simulink library "tqen"  (Simulink 8.2)
settings: Solver=ode45  SolverMode=SingleTasking  StartTime=0.0  StopTime=10.0  RelTol=1e-3
undefined symbols (not defined in the file or in its folder): ATQEN_BaseBrkDerateRatD_X_pct, ATQEN_BaseVehSpdRatD_X_kph, ATQEN_CruzAccLimIMult_X_mps2, ATQEN_CruzAccLimPMult_X_mps2, ATQEN_CruzContIMult_X_kph, ATQEN_CruzContPMult_X_kph, ATQEN_EngTqBrkMap_X_erpm, C_TASK_5MS_S, C_TICK_TIME_S, ENUM_ECMTQSOURCE_EXTERNAL, ENUM_ECMTQSOURCE_INTERNAL, ENUM_ECMTQSOURCE_TORQUELIM, ENUM_EMSHYBRIDOPSTATE_HYBRIDENABLE, ENUM_EMSOPSTATE_NORMAL, ENUM_GEARPOSN_PN, FALSE, KTQEN_AccelPedalFiltTm_s, KTQEN_BrakeSWTqDsblTimeThres_s, KTQEN_CruzAccLimErrGain_rat, KTQEN_CruzAccLimIGain_rat, KTQEN_CruzAccLimIMax_Nm, KTQEN_CruzAccLimIMin_Nm, KTQEN_CruzAccLimIRest_flg, KTQEN_CruzAccLimPGain_rat, KTQEN_CruzContAccLim_G, KTQEN_CruzContAccLimTqMax_Nm, KTQEN_CruzContAccLimTqMin_Nm, KTQEN_CruzContEnblSW_flg, KTQEN_CruzContErrGain_rat, KTQEN_CruzContIGain_rat, KTQEN_CruzContIMax_Nm, KTQEN_CruzContIMin_Nm, KTQEN_CruzContIRest_flg, KTQEN_CruzContPGain_rat, KTQEN_CruzContResumeSW_flg, KTQEN_CruzContSetSW_flg, KTQEN_CruzDsblDefaultTq_Nm, KTQEN_CruzSpdChgTimeThres_s, KTQEN_CruzTgSpdSetFalRate_kphps, KTQEN_CruzTgSpdSetRisRate_kphps, KTQEN_EngBrkTqMaxOvrd_Nm, KTQEN_EngBrkTqMinOvrd_Nm, KTQEN_VehAccCalRate_s, KTQEN_VehAccFltConst_s, KTQEN_VehSpdMaxVal_kph, KTQEN_VSGOVErrGain_rat, KTQEN_VSGOVIGain_rat, KTQEN_VSGOVIMax_Nm, KTQEN_VSGOVIMin_Nm, KTQEN_VSGOVIRest_flg, KTQEN_VSGOVMinVehSpd_kph, KTQEN_VSGOVPGain_rat, KTQEN_VSGOVTqDefault_Nm, KTQEN_VSGOVTqMax_Nm, KTQEN_VSGOVTqMin_Nm, MTQEN_BaseBrkDerateRatD_Y_pct, MTQEN_BasePedalSportMapHiSpdD_Z_pct, MTQEN_BasePedalSportMapLoSpdD_Z_pct, MTQEN_BaseTqSupptDeltPdlD_X_pctps, MTQEN_BaseTqSupptDeltPdlD_Y_pct ... (+9)
libraries: hcu_lib x6, tqen x3, simulink x1
(part 2 of 2)

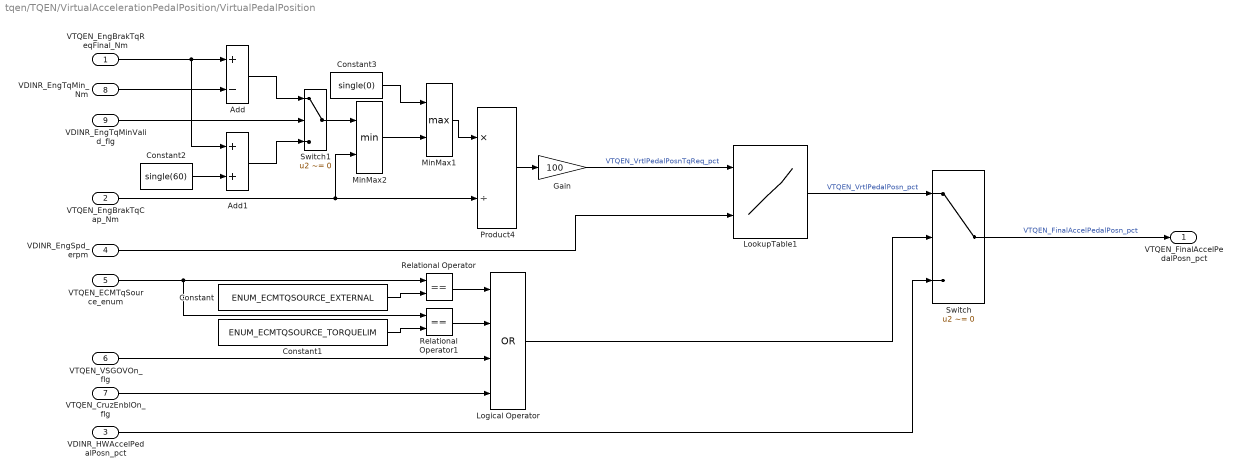
== system tqen/TQEN/VirtualAccelerationPedalPosition/VirtualPedalPosition ==
  VTQEN_EngBrakTqReqFinal_Nm : Inport
  VTQEN_EngBrakTqCap_Nm : Inport  Port=2
  VDINR_HWAccelPedalPosn_pct : Inport  Port=3
  VDINR_EngSpd_erpm : Inport  Port=4
  VTQEN_ECMTqSource_enum : Inport  Port=5
  VTQEN_VSGOVOn_flg : Inport  Port=6
  VTQEN_CruzEnblOn_flg : Inport  Port=7
  VDINR_EngTqMin_Nm : Inport  Port=8
  VDINR_EngTqMinValid_flg : Inport  Port=9
  Add : Sum  Inputs=+-
  Add1 : Sum
  Constant : Constant  Value=ENUM_ECMTQSOURCE_EXTERNAL
  Constant1 : Constant  Value=ENUM_ECMTQSOURCE_TORQUELIM
  Constant2 : Constant  Value=single(60)
  Constant3 : Constant  Value=single(0)
  Gain : Gain  Gain=100
  Logical Operator : Logic  Operator=OR  Inputs=4  AllPortsSameDT=off  OutDataTypeStr=boolean
  LookupTable1 : Lookup2D  RowIndex=ATQEN_VirtualPedalMap_X_pct  ColumnIndex=ATQEN_VirtualPedalMap_Y_erpm  Table=MTQEN_VirtualPedalMap_Z_pct  LookUpMeth=Interpolation-Use End Values
      settings: AttributesFormatString=<row =%<RowIndex>>\n<column = %<ColumnIndex>>\n<output = %<Table>>
  MinMax1 : MinMax  Function=max  Inputs=2
  MinMax2 : MinMax  Inputs=2
  Product4 : Product  Inputs=*/  RndMeth=Zero
  Relational Operator : RelationalOperator  Operator===  OutDataTypeStr=boolean
  Relational Operator1 : RelationalOperator  Operator===  OutDataTypeStr=boolean
  Switch : Switch  Criteria=u2 ~= 0
  Switch1 : Switch  Criteria=u2 ~= 0
  VTQEN_FinalAccelPedalPosn_pct : Outport
  wires:
  Constant3/1 -> MinMax1/1
  MinMax2/1 -> MinMax1/2
  Constant2/1 -> Add1/2
  VTQEN_EngBrakTqReqFinal_Nm/1 -> Add/1, Add1/1
  Add1/1 -> Switch1/3
  VDINR_EngTqMinValid_flg/1 -> Switch1/2
  Switch1/1 -> MinMax2/1
  VDINR_EngTqMin_Nm/1 -> Add/2
  Add/1 -> Switch1/1
  VTQEN_CruzEnblOn_flg/1 -> Logical Operator/4
  VTQEN_VSGOVOn_flg/1 -> Logical Operator/3
  Constant1/1 -> Relational Operator1/2
  Relational Operator1/1 -> Logical Operator/2
  Constant/1 -> Relational Operator/2
  Logical Operator/1 -> Switch/2
  LookupTable1/1 -> Switch/1  "VTQEN_VrtlPedalPosn_pct"
  VDINR_EngSpd_erpm/1 -> LookupTable1/2
  Relational Operator/1 -> Logical Operator/1
  Gain/1 -> LookupTable1/1  "VTQEN_VrtlPedalPosnTqReq_pct"
  Product4/1 -> Gain/1
  VTQEN_EngBrakTqCap_Nm/1 -> Product4/2, MinMax2/2
  MinMax1/1 -> Product4/1
  VDINR_HWAccelPedalPosn_pct/1 -> Switch/3
  VTQEN_ECMTqSource_enum/1 -> Relational Operator1/1, Relational Operator/1
  Switch/1 -> VTQEN_FinalAccelPedalPosn_pct/1  "VTQEN_FinalAccelPedalPosn_pct"

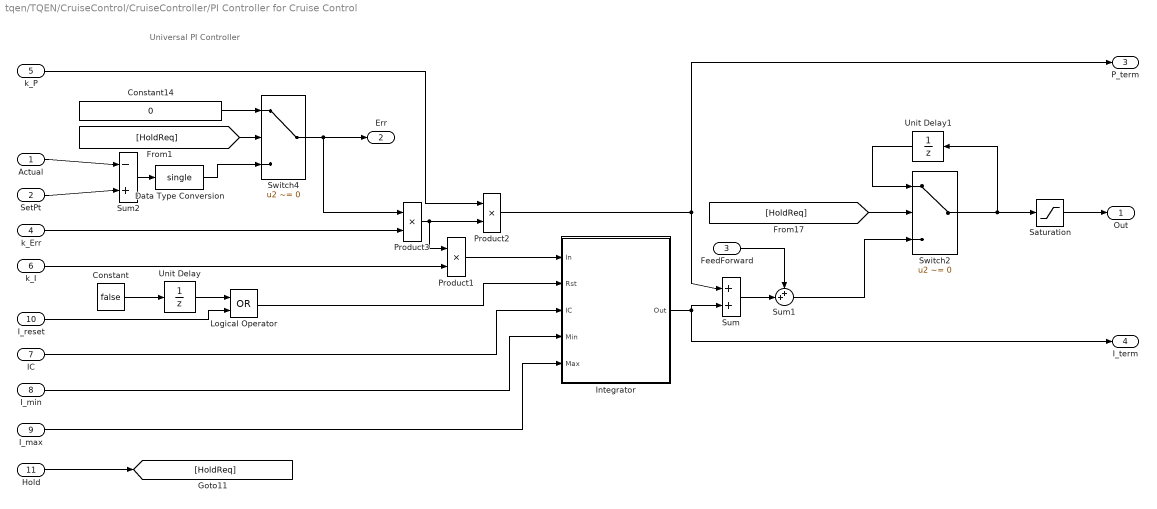
== system tqen/TQEN/CruiseControl/CruiseController/PI Controller for Cruise Control ==
  note: Universal PI Controller
  Actual : Inport
  SetPt : Inport  Port=2
  FeedForward : Inport  Port=3
  k_Err : Inport  Port=4
  k_P : Inport  Port=5
  k_I : Inport  Port=6
  IC : Inport  Port=7
  I_min : Inport  Port=8
  I_max : Inport  Port=9
  I_reset : Inport  Port=10
  Hold : Inport  Port=11
  Constant : Constant  Value=false  OutDataTypeStr=boolean
  Constant14 : Constant  Value=0  OutDataTypeStr=single
  Data Type Conversion : DataTypeConversion  OutDataTypeStr=single  SaturateOnIntegerOverflow=on  RndMeth=Zero
  Integrator : Subsystem  TreatAsAtomicUnit=on
  Logical Operator : Logic  Operator=OR  AllPortsSameDT=off  OutDataTypeStr=boolean
  Product1 : Product  InputSameDT=on  OutDataTypeStr=Inherit: Same as first input
  Product2 : Product  InputSameDT=on  OutDataTypeStr=Inherit: Same as first input
  Product3 : Product  InputSameDT=on  OutDataTypeStr=Inherit: Same as first input
  Saturation : Saturate  UpperLimit=inf  LowerLimit=0
  Sum : Sum  Inputs=+|+  SaturateOnIntegerOverflow=on  InputSameDT=on  OutDataTypeStr=Inherit: Same as first input
  Sum1 : Sum  Inputs=++|
  Sum2 : Sum  Inputs=-|+  SaturateOnIntegerOverflow=on  InputSameDT=on  OutDataTypeStr=Inherit: Same as first input
  Switch2 : Switch  Criteria=u2 ~= 0
  Switch4 : Switch  Criteria=u2 ~= 0
  Unit Delay : UnitDelay  InitialCondition=true  SampleTime=-1
  Unit Delay1 : UnitDelay  SampleTime=-1
  Out : Outport  OutputWhenDisabled=reset  InitialOutput=[0]
  Err : Outport  Port=2  OutputWhenDisabled=reset  InitialOutput=[0]
  P_term : Outport  Port=3  OutputWhenDisabled=reset  InitialOutput=[0]
  I_term : Outport  Port=4  OutputWhenDisabled=reset  InitialOutput=[0]
  wires:
  I_max/1 -> Integrator/5(Max)
  I_min/1 -> Integrator/4(Min)
  k_Err/1 -> Product3/2
  SetPt/1 -> Sum2/2
  Actual/1 -> Sum2/1
  k_P/1 -> Product2/1
  k_I/1 -> Product1/2
  Product1/1 -> Integrator/1(In)
  Product2/1 -> P_term/1, Sum/1
  Integrator/1(Out) -> I_term/1, Sum/2
  Sum/1 -> Sum1/2
  IC/1 -> Integrator/3(IC)
  Product3/1 -> Product2/2, Product1/1
  Sum2/1 -> Data Type Conversion/1
  Logical Operator/1 -> Integrator/2(Rst)
  I_reset/1 -> Logical Operator/2
  Unit Delay/1 -> Logical Operator/1
  Constant/1 -> Unit Delay/1
  Hold/1 -> [HoldReq]
  [HoldReq] -> Switch2/2
  Switch2/1 -> Unit Delay1/1, Saturation/1
  Unit Delay1/1 -> Switch2/1
  Switch4/1 -> Err/1, Product3/1
  Data Type Conversion/1 -> Switch4/3
  [HoldReq] -> Switch4/2
  Constant14/1 -> Switch4/1
  Sum1/1 -> Switch2/3
  FeedForward/1 -> Sum1/1
  Saturation/1 -> Out/1

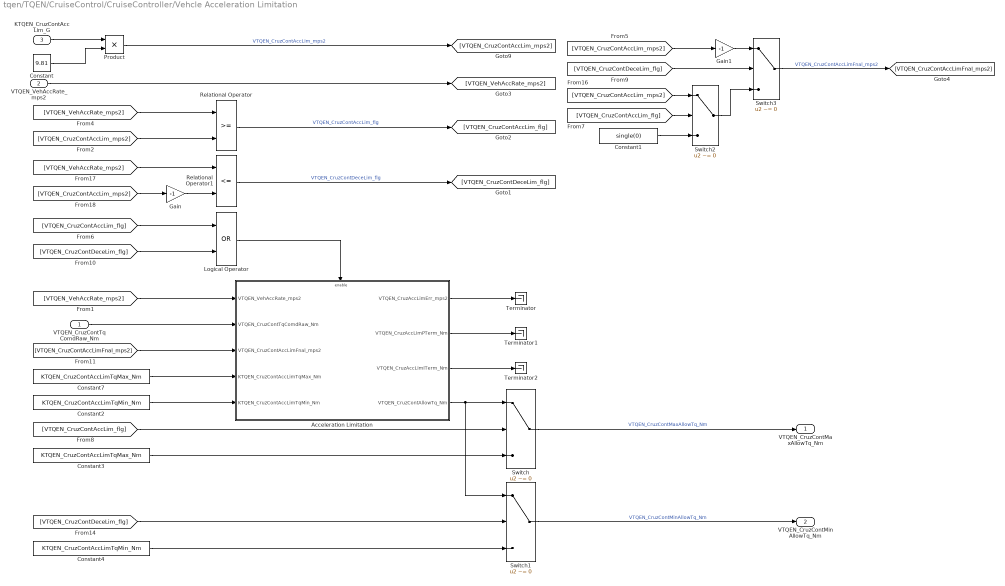
== system tqen/TQEN/CruiseControl/CruiseController/Vehcle Acceleration Limitation ==
  VTQEN_CruzContTqComdRaw_Nm : Inport
  VTQEN_VehAccRate_mps2 : Inport  Port=2
  KTQEN_CruzContAccLim_G : Inport  Port=3
  Acceleration Limitation : Subsystem  TreatAsAtomicUnit=on
  Constant : Constant  Value=9.81  OutDataTypeStr=single
  Constant1 : Constant  Value=single(0)
  Constant2 : Constant  Value=KTQEN_CruzContAccLimTqMin_Nm
  Constant3 : Constant  Value=KTQEN_CruzContAccLimTqMax_Nm
  Constant4 : Constant  Value=KTQEN_CruzContAccLimTqMin_Nm
  Constant7 : Constant  Value=KTQEN_CruzContAccLimTqMax_Nm
  Gain : Gain  Gain=-1
  Gain1 : Gain  Gain=-1
  Logical Operator : Logic  Operator=OR  AllPortsSameDT=off  OutDataTypeStr=boolean
  Product : Product  RndMeth=Zero
  Relational Operator : RelationalOperator  OutDataTypeStr=boolean
  Relational Operator1 : RelationalOperator  Operator=<=  OutDataTypeStr=boolean
  Switch{,1..3} (4 alike) : Switch  Criteria=u2 ~= 0
  Terminator : Terminator
  Terminator1 : Terminator
  Terminator2 : Terminator
  VTQEN_CruzContMaxAllowTq_Nm : Outport
  VTQEN_CruzContMinAllowTq_Nm : Outport  Port=2
  wires:
  Acceleration Limitation/3(VTQEN_CruzAccLimITerm_Nm) -> Terminator2/1
  Acceleration Limitation/2(VTQEN_CruzAccLimPTerm_Nm) -> Terminator1/1
  Constant2/1 -> Acceleration Limitation/5(KTQEN_CruzContAccLimTqMin_Nm)
  [VTQEN_CruzContDeceLim_flg] -> Logical Operator/2
  [VTQEN_CruzContAccLim_flg] -> Logical Operator/1
  Switch3/1 -> [VTQEN_CruzContAccLimFnal_mps2]  "VTQEN_CruzContAccLimFnal_mps2"
  Gain1/1 -> Switch3/1
  [VTQEN_CruzContAccLim_mps2] -> Gain1/1
  Switch2/1 -> Switch3/3
  [VTQEN_CruzContDeceLim_flg] -> Switch3/2
  Constant1/1 -> Switch2/3
  [VTQEN_CruzContAccLim_mps2] -> Switch2/1
  [VTQEN_CruzContAccLim_flg] -> Switch2/2
  Constant7/1 -> Acceleration Limitation/4(KTQEN_CruzContAccLimTqMax_Nm)
  [VTQEN_CruzContDeceLim_flg] -> Switch1/2
  [VTQEN_CruzContAccLim_flg] -> Switch/2
  Constant4/1 -> Switch1/3
  Switch1/1 -> VTQEN_CruzContMinAllowTq_Nm/1  "VTQEN_CruzContMinAllowTq_Nm"
  Gain/1 -> Relational Operator1/2
  Relational Operator1/1 -> [VTQEN_CruzContDeceLim_flg]  "VTQEN_CruzContDeceLim_flg"
  [VTQEN_CruzContAccLim_mps2] -> Gain/1
  [VTQEN_VehAccRate_mps2] -> Relational Operator1/1
  Relational Operator/1 -> [VTQEN_CruzContAccLim_flg]  "VTQEN_CruzContAccLim_flg"
  [VTQEN_CruzContAccLim_mps2] -> Relational Operator/2
  [VTQEN_VehAccRate_mps2] -> Relational Operator/1
  VTQEN_VehAccRate_mps2/1 -> [VTQEN_VehAccRate_mps2]
  Constant/1 -> Product/2
  KTQEN_CruzContAccLim_G/1 -> Product/1
  Product/1 -> [VTQEN_CruzContAccLim_mps2]  "VTQEN_CruzContAccLim_mps2"
  Logical Operator/1 -> Acceleration Limitation/Enable
  Constant3/1 -> Switch/3
  Acceleration Limitation/4(VTQEN_CruzContAllowTq_Nm) -> Switch1/1, Switch/1
  [VTQEN_VehAccRate_mps2] -> Acceleration Limitation/1(VTQEN_VehAccRate_mps2)
  VTQEN_CruzContTqComdRaw_Nm/1 -> Acceleration Limitation/2(VTQEN_CruzContTqComdRaw_Nm)
  [VTQEN_CruzContAccLimFnal_mps2] -> Acceleration Limitation/3(VTQEN_CruzContAccLimFnal_mps2)
  Switch/1 -> VTQEN_CruzContMaxAllowTq_Nm/1  "VTQEN_CruzContMaxAllowTq_Nm"
  Acceleration Limitation/1(VTQEN_CruzAccLimErr_mps2) -> Terminator/1

== system tqen/TQEN/CruiseControl/Rate_Limit/RateLimiter ==
  Data_Input : Inport
  Rising Rate : Inport  Port=2
  Falling Rate : Inport  Port=3
  Initial_Condition : Inport  Port=4
  Chart : Stateflow chart  TreatAsAtomicUnit=on
  Constant : Constant  Value=C_TICK_TIME_S
  Constant1 : Constant  Value=C_TICK_TIME_S
  Constant2 : Constant  Value=single(1)
  Constant4 : Constant  Value=single(1)
  Data Type Conversion : DataTypeConversion  OutDataTypeStr=boolean
  Data Type Conversion1 : DataTypeConversion  OutDataTypeStr=boolean
  Product{1..4} (4 alike) : Product  Inputs=*/  RndMeth=Zero
  Relational Operator : RelationalOperator  Operator=>  OutDataTypeStr=boolean
  Relational Operator1 : RelationalOperator  Operator=<  OutDataTypeStr=boolean
  Saturation : Subsystem
  Sum1 : Sum  Inputs=|++
  Switch1 : Switch  Threshold=0.5
  Unit Delay1 : UnitDelay  SampleTime=-1
  Data_Output : Outport
  wires:
  Constant2/1 -> Product4/1
  Unit Delay1/1 -> Relational Operator1/2, Relational Operator/2, Sum1/2
  Sum1/1 -> Saturation/1(in)
  Falling Rate/1 -> Product2/1
  Rising Rate/1 -> Product1/1
  Switch1/1 -> Unit Delay1/1, Data_Output/1
  Constant1/1 -> Product4/2
  Constant4/1 -> Product3/1
  Constant/1 -> Product3/2
  Initial_Condition/1 -> Switch1/1
  Chart/1(Initial) -> Switch1/2
  Chart/4(Max) -> Saturation/3(max)
  Chart/3(Min) -> Saturation/2(min)
  Saturation/1(out) -> Switch1/3
  Chart/2(tou) -> Sum1/1
  Data Type Conversion1/1 -> Chart/1(increase)
  Data Type Conversion/1 -> Chart/2(decrease)
  Product2/1 -> Chart/5(decrease_tou)
  Product1/1 -> Chart/4(increase_tou)
  Product4/1 -> Product2/2
  Product3/1 -> Product1/2
  Data_Input/1 -> Chart/3(Data_in), Relational Operator1/1, Relational Operator/1
  Relational Operator/1 -> Data Type Conversion1/1
  Relational Operator1/1 -> Data Type Conversion/1

== system tqen/TQEN/CruiseControl/Trigger signal generator/trigger signal generator ==
  Time_dur [s] : Inport
  Constant3 : Constant  Value=0  OutDataTypeStr=single
  Constant4 : Constant  Value=C_TICK_TIME_S
  Relational Operator1 : RelationalOperator  OutDataTypeStr=boolean
  Sum1 : Sum  Inputs=|++  SaturateOnIntegerOverflow=on  InputSameDT=on
  Sum2 : Sum  Inputs=+-
  Switch3 : Switch  Threshold=0.5
  Unit Delay2 : UnitDelay  SampleTime=-1
  Unit Delay3 : UnitDelay  SampleTime=-1
  Trigger_signal : Outport  OutputWhenDisabled=reset  InitialOutput=[0]
  wires:
  Sum2/1 -> Relational Operator1/2
  Unit Delay3/1 -> Switch3/2
  Unit Delay2/1 -> Sum1/2
  Switch3/1 -> Relational Operator1/1, Unit Delay2/1
  Constant3/1 -> Switch3/1
  Time_dur [s]/1 -> Sum2/1
  Relational Operator1/1 -> Unit Delay3/1, Trigger_signal/1
  Constant4/1 -> Sum2/2, Sum1/1
  Sum1/1 -> Switch3/3

== system tqen/TQEN/CruiseControl/Vehicle Acceleration Calculation/signal_filter ==
  raw_input : Inport
  Tc : Inport  Port=2
  Ts : Inport  Port=3
  FirstOrderFilter : hcu_lib/FirstOrderFilter  SystemSampleTime=-1
  IC : UnitDelay  Tag=struct('comment',struct('text','','placement',1),'logdata',struct('maxnumvals',inf,'plotchannels',[],'stepsize',0,'downsampling',1,'loggingmode',3,'channels',1),'output',struct('width',1,'name','$S_$B','unit','','type','Int16','offset',0,'max',NaN,'min',NaN,'freeze',1,'lsb',1,'arb',0,'class','default','address','','description','','autoscalingmode',1,'lowerheadroom',1,'upperheadroom',1,'headroomunit','bit','checkmin',0,'checkmax',0,'show',0,'initial','2'),'state',0,'dt','-1','date',731455.586925799)  SampleTime=-1
  Switch1 : Switch  Tag=struct('comment',struct('text','','placement',1),'logdata',struct('maxnumvals',inf,'plotchannels',[],'stepsize',0,'downsampling',1,'loggingmode',3,'channels',1),'output',struct('width',1,'name','$S_$B','unit','','type','Int32Bin15','offset',0,'max',65535,'min',-65536,'freeze',1,'lsb',2^-15,'arb',0,'class','default','address','','description','','autoscalingmode',1,'lowerheadroom',1,'upperheadroom',1,'headroomunit','bit','checkmin',0,'checkmax',0,'show',0),'threshold',struct('width',1,'name','$S_$B_threshold','unit','','type','Int16','offset',0,'max',NaN,'min',NaN,'freeze',1,'lsb',1,'arb',0,'class','default','address','','description','','value','1','scalar',0),'date',731455.58657044)  Threshold=0.5  InputSameDT=on
  zero : Constant  Tag=struct('comment',struct('text','','placement',1),'output',struct('width',1,'name','$S_$B','unit','','type','Int16','offset',0,'max',NaN,'min',NaN,'freeze',1,'lsb',1,'arb',0,'class','default','address','','description','','value','0','tolerance',1,'show',0),'date',731455.58675544)  Value=TRUE
  zero1 : Constant  Tag=struct('comment',struct('text','','placement',1),'output',struct('width',1,'name','$S_$B','unit','','type','Int16','offset',0,'max',NaN,'min',NaN,'freeze',1,'lsb',1,'arb',0,'class','default','address','','description','','value','0','tolerance',1,'show',0),'date',731455.58675544)  Value=0  OutDataTypeStr=single
  raw_input_filt : Outport
  wires:
  zero/1 -> IC/1
  raw_input/1 -> FirstOrderFilter/1
  Tc/1 -> Switch1/1
  Ts/1 -> FirstOrderFilter/3
  IC/1 -> Switch1/2
  FirstOrderFilter/1 -> raw_input_filt/1
  Switch1/1 -> FirstOrderFilter/2
  zero1/1 -> Switch1/3

== system tqen/TQEN/Governor/Vehcle Speed Governing/Vehicle Speed Governor ==
  VDINR_VehSpd_kph : Inport
  VTQEN_EngBrakTqReqRaw_Nm : Inport  Port=2
  VTQEN_VehSpdLimVal_kph : Inport  Port=3
  Enable : EnablePort  StatesWhenEnabling=reset
  Constant1 : Constant  Value=FALSE
  Constant11 : Constant  Value=KTQEN_VSGOVIMax_Nm
  Constant12 : Constant  Value=KTQEN_VSGOVIMin_Nm
  Constant13 : Constant  Value=KTQEN_VSGOVIRest_flg
  Constant2 : Constant  Value=single(0)
  Constant3 : Constant  Value=KTQEN_VSGOVTqMax_Nm
  Constant4 : Constant  Value=KTQEN_VSGOVTqMin_Nm
  Constant7 : Constant  Value=KTQEN_VSGOVErrGain_rat
  Constant8 : Constant  Value=KTQEN_VSGOVPGain_rat
  Constant9 : Constant  Value=KTQEN_VSGOVIGain_rat
  Limit : hcu_lib/Limit  SystemSampleTime=-1
  PI Controller for Vehicle Governor : Subsystem  TreatAsAtomicUnit=on
  VTQEN_VSGOVErr_kph : Outport  OutputWhenDisabled=reset  InitialOutput=[0]
  VTQEN_VSGOVPTerm_Nm : Outport  Port=2  OutputWhenDisabled=reset  InitialOutput=[0]
  VTQEN_VSGOVITerm_Nm : Outport  Port=3  OutputWhenDisabled=reset  InitialOutput=[0]
  VTQEN_VSGOVTqComd_Nm : Outport  Port=4  OutputWhenDisabled=reset  InitialOutput=[0]
  wires:
  Constant4/1 -> Limit/3
  Constant3/1 -> Limit/2
  Limit/1 -> VTQEN_VSGOVTqComd_Nm/1  "VTQEN_VSGOVTqComd_Nm"
  Constant2/1 -> PI Controller for Vehicle Governor/3(FeedForward)
  Constant1/1 -> PI Controller for Vehicle Governor/11(Hold)
  Constant9/1 -> PI Controller for Vehicle Governor/6(k_I)
  PI Controller for Vehicle Governor/4(I_term) -> VTQEN_VSGOVITerm_Nm/1  "VTQEN_VSGOVITerm_Nm"
  PI Controller for Vehicle Governor/3(P_term) -> VTQEN_VSGOVPTerm_Nm/1  "VTQEN_VSGOVPTerm_Nm"
  PI Controller for Vehicle Governor/2(Err) -> VTQEN_VSGOVErr_kph/1  "VTQEN_VSGOVErr_kph"
  Constant13/1 -> PI Controller for Vehicle Governor/10(I_reset)
  Constant11/1 -> PI Controller for Vehicle Governor/9(I_max)
  Constant12/1 -> PI Controller for Vehicle Governor/8(I_min)
  VTQEN_EngBrakTqReqRaw_Nm/1 -> PI Controller for Vehicle Governor/7(IC)
  Constant8/1 -> PI Controller for Vehicle Governor/5(k_P)
  Constant7/1 -> PI Controller for Vehicle Governor/4(k_Err)
  VTQEN_VehSpdLimVal_kph/1 -> PI Controller for Vehicle Governor/2(SetPt)
  VDINR_VehSpd_kph/1 -> PI Controller for Vehicle Governor/1(Actual)
  PI Controller for Vehicle Governor/1(Out) -> Limit/1  "VTQEN_VSGOVTqComdRaw_Nm"

== system tqen/TQEN/PedalTorqueDemand/PedalTorqueDemandCalculation/PedalFeelMap ==
  VDINR_HWAccelPedalPosn_pct : Inport
  VDINR_EngSpd_erpm : Inport  Port=2
  PedalMap : Subsystem  TreatAsAtomicUnit=on
  VTQEN_PedalTqSportLoD_pct : Outport
  VTQEN_PedalTqSportlHiD_pct : Outport  Port=2
  wires:
  PedalMap/2(VTQEN_PedalTqSportlHiD_pct) -> VTQEN_PedalTqSportlHiD_pct/1
  PedalMap/1(VTQEN_PedalTqSportLoD_pct) -> VTQEN_PedalTqSportLoD_pct/1
  VDINR_EngSpd_erpm/1 -> PedalMap/2(VDINR_EngSpd_erpm)
  VDINR_HWAccelPedalPosn_pct/1 -> PedalMap/1(VDINR_HWAccelPedalPosn_pct)

== system tqen/TQEN/PedalTorqueDemand/PedalTorqueDemandCalculation/PedalTorqueCalculation ==
  task_time_s : Inport
  VDINR_HWAccelPedalPosn_pct : Inport  Port=2
  VTQEN_PedalTqSportLoD_pct : Inport  Port=3
  VTQEN_PedalTqSportlHiD_pct : Inport  Port=4
  VDINR_VehSpd_kph : Inport  Port=5
  VTQEN_EngBrakTqCap_Nm : Inport  Port=6
  VDINR_BrkLampOn_flg : Inport  Port=7
  Constant : Constant  OutDataTypeStr=single
  Constant2 : Constant  Value=100  OutDataTypeStr=single
  Data Type Conversion : DataTypeConversion  OutDataTypeStr=single
  Gain : Gain  Gain=0.01
  Gain1 : Gain  Gain=0.01
  Gain2 : Gain  Gain=0.01
  Lookup Table : Lookup  InputValues=ATQEN_BaseVehSpdRatD_X_kph  Table=MTQEN_BaseVehSpdRatD_Y_pct  LookUpMeth=Interpolation-Use End Values
      settings: AttributesFormatString=<input =%<InputValues>>\n<output = %<Table>>
  Lookup Table1 : Lookup  InputValues=ATQEN_BaseBrkDerateRatD_X_pct  Table=MTQEN_BaseBrkDerateRatD_Y_pct  LookUpMeth=Interpolation-Use End Values
      settings: AttributesFormatString=<input =%<InputValues>>\n<output = %<Table>>
  Product{,1..3} (4 alike) : Product  RndMeth=Zero
  Product4 : Product  OutDataTypeStr=single  RndMeth=Zero
  Saturation : Saturate  UpperLimit=100  LowerLimit=0
      settings: AttributesFormatString=<%<LowerLimit>->%<UpperLimit>>
  Subtract : Sum  Inputs=+-
  Subtract1 : Sum  Inputs=+++
  TqSupport4QuickPedalChange : Subsystem
  VTQEN_PedalTqDem_Nm : Outport
  wires:
  VTQEN_EngBrakTqCap_Nm/1 -> Product3/2
  Product3/1 -> VTQEN_PedalTqDem_Nm/1  "VTQEN_PedalTqDem_Nm"
  VDINR_VehSpd_kph/1 -> Lookup Table/1
  Product2/1 -> Gain2/1  "VTQEN_PedalTqDemReduced_pct"
  Gain1/1 -> Product2/2
  Lookup Table1/1 -> Gain1/1  "VTQEN_PedalTqDemBrakReduce_pct"
  Subtract1/1 -> Saturation/1
  Product1/1 -> Subtract1/2
  Product/1 -> Subtract1/1
  Constant/1 -> Subtract/1
  Subtract/1 -> Product1/1
  VTQEN_PedalTqSportlHiD_pct/1 -> Product1/2
  Gain/1 -> Subtract/2, Product/2
  VTQEN_PedalTqSportLoD_pct/1 -> Product/1
  Lookup Table/1 -> Gain/1  "VTQEN_BaseVehSpdRatD_pct"
  Gain2/1 -> Product3/1
  VDINR_BrkLampOn_flg/1 -> Data Type Conversion/1
  Product4/1 -> Lookup Table1/1
  VDINR_HWAccelPedalPosn_pct/1 -> TqSupport4QuickPedalChange/1(VDINR_HWAccelPedalPosn_pct)
  TqSupport4QuickPedalChange/1(VTQEN_DeltPedalComp_pct) -> Subtract1/3
  task_time_s/1 -> TqSupport4QuickPedalChange/2(task_time_s)
  Constant2/1 -> Product4/2
  Data Type Conversion/1 -> Product4/1
  Saturation/1 -> Product2/1  "VTQEN_PedalTqDemRaw_pct"

== system tqen/TQEN/CruiseControl/CruiseController/PI Controller for Cruise Control/Integrator ==
  In : Inport
  Rst : Inport  Port=2
  IC : Inport  Port=3
  Min : Inport  Port=4
  Max : Inport  Port=5
  Constant : Constant  Value=C_TICK_TIME_S  OutDataTypeStr=single
  Data Type Conversion : DataTypeConversion  OutDataTypeStr=boolean  RndMeth=Zero
  Product : Product  SaturateOnIntegerOverflow=on  InputSameDT=on  OutDataTypeStr=Inherit: Same as first input
  Saturation : Subsystem
  Sum : Sum  Inputs=++|  SaturateOnIntegerOverflow=on  InputSameDT=on
  Switch1 : Switch  Threshold=1  ZeroCross=off  SaturateOnIntegerOverflow=on  InputSameDT=on
  Unit Delay : UnitDelay  SampleTime=-1
  Out : Outport
  wires:
  Saturation/1(out) -> Unit Delay/1
  Sum/1 -> Saturation/1(in)
  Switch1/1 -> Out/1, Sum/1
  Constant/1 -> Product/2
  In/1 -> Product/1
  Product/1 -> Sum/2
  Unit Delay/1 -> Switch1/3
  Rst/1 -> Data Type Conversion/1
  Data Type Conversion/1 -> Switch1/2
  Min/1 -> Saturation/2(min)
  Max/1 -> Saturation/3(max)
  IC/1 -> Switch1/1

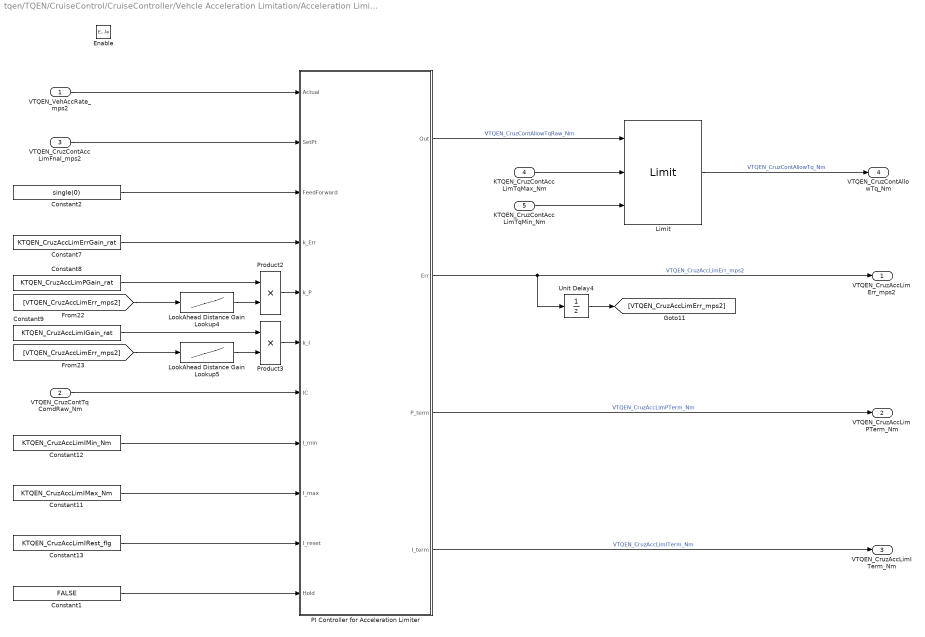
== system tqen/TQEN/CruiseControl/CruiseController/Vehcle Acceleration Limitation/Acceleration Limitation ==
  VTQEN_VehAccRate_mps2 : Inport
  VTQEN_CruzContTqComdRaw_Nm : Inport  Port=2
  VTQEN_CruzContAccLimFnal_mps2 : Inport  Port=3
  KTQEN_CruzContAccLimTqMax_Nm : Inport  Port=4
  KTQEN_CruzContAccLimTqMin_Nm : Inport  Port=5
  Enable : EnablePort  StatesWhenEnabling=reset
  Constant1 : Constant  Value=FALSE
  Constant11 : Constant  Value=KTQEN_CruzAccLimIMax_Nm
  Constant12 : Constant  Value=KTQEN_CruzAccLimIMin_Nm
  Constant13 : Constant  Value=KTQEN_CruzAccLimIRest_flg
  Constant2 : Constant  Value=single(0)
  Constant7 : Constant  Value=KTQEN_CruzAccLimErrGain_rat
  Constant8 : Constant  Value=KTQEN_CruzAccLimPGain_rat
  Constant9 : Constant  Value=KTQEN_CruzAccLimIGain_rat
  Limit : hcu_lib/Limit  SystemSampleTime=-1
  LookAhead Distance Gain Lookup4 : Lookup  InputValues=ATQEN_CruzAccLimPMult_X_mps2  Table=MTQEN_CruzAccLimPMult_rat  LookUpMeth=Interpolation-Use End Values
      settings: AttributesFormatString=%<InputValues>\n%<Table>
  LookAhead Distance Gain Lookup5 : Lookup  InputValues=ATQEN_CruzAccLimIMult_X_mps2  Table=MTQEN_CruzAccLimIMult_rat  LookUpMeth=Interpolation-Use End Values
      settings: AttributesFormatString=%<InputValues>\n%<Table>
  PI Controller for Acceleration Limiter : Subsystem  TreatAsAtomicUnit=on
  Product2 : Product  OutDataTypeStr=single  RndMeth=Zero
  Product3 : Product  OutDataTypeStr=single  RndMeth=Zero
  Unit Delay4 : UnitDelay  SampleTime=-1
  VTQEN_CruzAccLimErr_mps2 : Outport  OutputWhenDisabled=reset  InitialOutput=[0]
  VTQEN_CruzAccLimPTerm_Nm : Outport  Port=2  OutputWhenDisabled=reset  InitialOutput=[0]
  VTQEN_CruzAccLimITerm_Nm : Outport  Port=3  OutputWhenDisabled=reset  InitialOutput=[0]
  VTQEN_CruzContAllowTq_Nm : Outport  Port=4  OutputWhenDisabled=reset  InitialOutput=[0]
  wires:
  PI Controller for Acceleration Limiter/1(Out) -> Limit/1  "VTQEN_CruzContAllowTqRaw_Nm"
  Limit/1 -> VTQEN_CruzContAllowTq_Nm/1  "VTQEN_CruzContAllowTq_Nm"
  KTQEN_CruzContAccLimTqMax_Nm/1 -> Limit/2
  KTQEN_CruzContAccLimTqMin_Nm/1 -> Limit/3
  Constant2/1 -> PI Controller for Acceleration Limiter/3(FeedForward)
  Constant1/1 -> PI Controller for Acceleration Limiter/11(Hold)
  Unit Delay4/1 -> [VTQEN_CruzAccLimErr_mps2]
  [VTQEN_CruzAccLimErr_mps2] -> LookAhead Distance Gain Lookup5/1
  Constant9/1 -> Product3/1
  Product3/1 -> PI Controller for Acceleration Limiter/6(k_I)
  LookAhead Distance Gain Lookup5/1 -> Product3/2
  [VTQEN_CruzAccLimErr_mps2] -> LookAhead Distance Gain Lookup4/1
  LookAhead Distance Gain Lookup4/1 -> Product2/2
  Product2/1 -> PI Controller for Acceleration Limiter/5(k_P)
  PI Controller for Acceleration Limiter/4(I_term) -> VTQEN_CruzAccLimITerm_Nm/1  "VTQEN_CruzAccLimITerm_Nm"
  PI Controller for Acceleration Limiter/3(P_term) -> VTQEN_CruzAccLimPTerm_Nm/1  "VTQEN_CruzAccLimPTerm_Nm"
  PI Controller for Acceleration Limiter/2(Err) -> VTQEN_CruzAccLimErr_mps2/1, Unit Delay4/1  "VTQEN_CruzAccLimErr_mps2"
  Constant13/1 -> PI Controller for Acceleration Limiter/10(I_reset)
  Constant11/1 -> PI Controller for Acceleration Limiter/9(I_max)
  Constant12/1 -> PI Controller for Acceleration Limiter/8(I_min)
  VTQEN_CruzContTqComdRaw_Nm/1 -> PI Controller for Acceleration Limiter/7(IC)
  Constant8/1 -> Product2/1
  Constant7/1 -> PI Controller for Acceleration Limiter/4(k_Err)
  VTQEN_CruzContAccLimFnal_mps2/1 -> PI Controller for Acceleration Limiter/2(SetPt)
  VTQEN_VehAccRate_mps2/1 -> PI Controller for Acceleration Limiter/1(Actual)

== system tqen/TQEN/CruiseControl/Rate_Limit/RateLimiter/Saturation ==
  in : Inport
  min : Inport  Port=2
  max : Inport  Port=3
  MinMax : MinMax  Function=max  Inputs=2  ZeroCross=off  SaturateOnIntegerOverflow=on  InputSameDT=on
  MinMax1 : MinMax  Inputs=2  ZeroCross=off  SaturateOnIntegerOverflow=on  InputSameDT=on
  out : Outport
  wires:
  MinMax/1 -> MinMax1/1
  in/1 -> MinMax/1
  min/1 -> MinMax/2
  max/1 -> MinMax1/2
  MinMax1/1 -> out/1

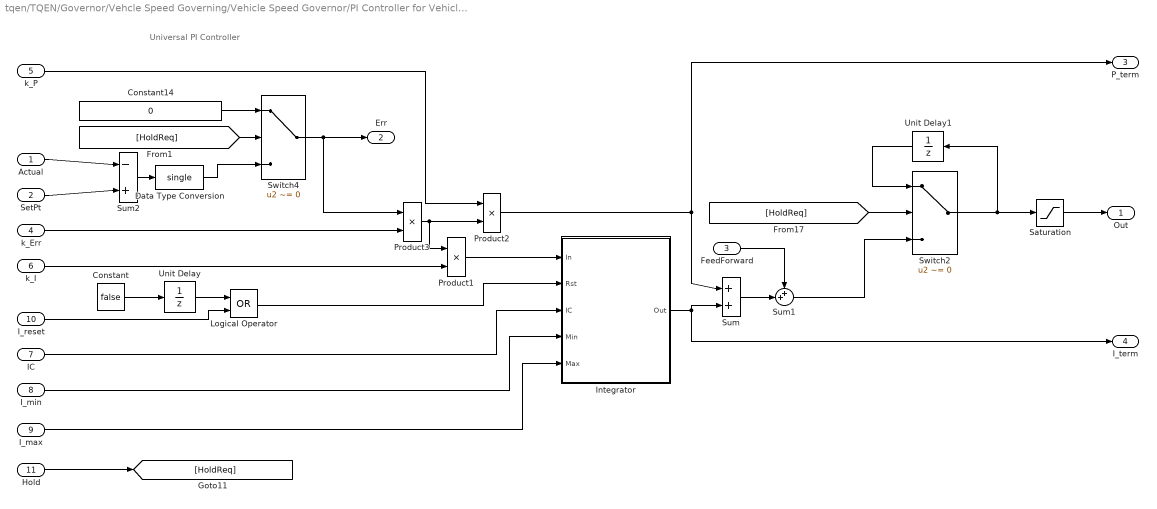
== system tqen/TQEN/Governor/Vehcle Speed Governing/Vehicle Speed Governor/PI Controller for Vehicle Governor ==
  note: Universal PI Controller
  Actual : Inport
  SetPt : Inport  Port=2
  FeedForward : Inport  Port=3
  k_Err : Inport  Port=4
  k_P : Inport  Port=5
  k_I : Inport  Port=6
  IC : Inport  Port=7
  I_min : Inport  Port=8
  I_max : Inport  Port=9
  I_reset : Inport  Port=10
  Hold : Inport  Port=11
  Constant : Constant  Value=false  OutDataTypeStr=boolean
  Constant14 : Constant  Value=0  OutDataTypeStr=single
  Data Type Conversion : DataTypeConversion  OutDataTypeStr=single  SaturateOnIntegerOverflow=on  RndMeth=Zero
  Integrator : Subsystem  TreatAsAtomicUnit=on
  Logical Operator : Logic  Operator=OR  AllPortsSameDT=off  OutDataTypeStr=boolean
  Product1 : Product  InputSameDT=on  OutDataTypeStr=Inherit: Same as first input
  Product2 : Product  InputSameDT=on  OutDataTypeStr=Inherit: Same as first input
  Product3 : Product  InputSameDT=on  OutDataTypeStr=Inherit: Same as first input
  Saturation : Saturate  UpperLimit=inf  LowerLimit=0
  Sum : Sum  Inputs=+|+  SaturateOnIntegerOverflow=on  InputSameDT=on  OutDataTypeStr=Inherit: Same as first input
  Sum1 : Sum  Inputs=++|
  Sum2 : Sum  Inputs=-|+  SaturateOnIntegerOverflow=on  InputSameDT=on  OutDataTypeStr=Inherit: Same as first input
  Switch2 : Switch  Criteria=u2 ~= 0
  Switch4 : Switch  Criteria=u2 ~= 0
  Unit Delay : UnitDelay  InitialCondition=true  SampleTime=-1
  Unit Delay1 : UnitDelay  SampleTime=-1
  Out : Outport  OutputWhenDisabled=reset  InitialOutput=[0]
  Err : Outport  Port=2  OutputWhenDisabled=reset  InitialOutput=[0]
  P_term : Outport  Port=3  OutputWhenDisabled=reset  InitialOutput=[0]
  I_term : Outport  Port=4  OutputWhenDisabled=reset  InitialOutput=[0]
  wires:
  I_max/1 -> Integrator/5(Max)
  I_min/1 -> Integrator/4(Min)
  k_Err/1 -> Product3/2
  SetPt/1 -> Sum2/2
  Actual/1 -> Sum2/1
  k_P/1 -> Product2/1
  k_I/1 -> Product1/2
  Product1/1 -> Integrator/1(In)
  Product2/1 -> P_term/1, Sum/1
  Integrator/1(Out) -> I_term/1, Sum/2
  Sum/1 -> Sum1/2
  IC/1 -> Integrator/3(IC)
  Product3/1 -> Product2/2, Product1/1
  Sum2/1 -> Data Type Conversion/1
  Logical Operator/1 -> Integrator/2(Rst)
  I_reset/1 -> Logical Operator/2
  Unit Delay/1 -> Logical Operator/1
  Constant/1 -> Unit Delay/1
  Hold/1 -> [HoldReq]
  [HoldReq] -> Switch2/2
  Switch2/1 -> Unit Delay1/1, Saturation/1
  Unit Delay1/1 -> Switch2/1
  Switch4/1 -> Err/1, Product3/1
  Data Type Conversion/1 -> Switch4/3
  [HoldReq] -> Switch4/2
  Constant14/1 -> Switch4/1
  Sum1/1 -> Switch2/3
  FeedForward/1 -> Sum1/1
  Saturation/1 -> Out/1

== system tqen/TQEN/PedalTorqueDemand/PedalTorqueDemandCalculation/PedalFeelMap/PedalMap ==
  VDINR_HWAccelPedalPosn_pct : Inport
  VDINR_EngSpd_erpm : Inport  Port=2
  LookupTable : Lookup2D  RowIndex=ATQEN_BasePedalMapLoSpdD_X_pct  ColumnIndex=ATQEN_BasePedalMapLoSpdD_Y_erpm  Table=MTQEN_BasePedalSportMapLoSpdD_Z_pct  LookUpMeth=Interpolation-Use End Values
      settings: AttributesFormatString=<row =%<RowIndex>>\n<column = %<ColumnIndex>>\n<output = %<Table>>
  LookupTable1 : Lookup2D  RowIndex=ATQEN_BasePedalMapHiSpdD_X_pct  ColumnIndex=ATQEN_BasePedalMapHiSpdD_Y_erpm  Table=MTQEN_BasePedalSportMapHiSpdD_Z_pct  LookUpMeth=Interpolation-Use End Values
      settings: AttributesFormatString=<row =%<RowIndex>>\n<column = %<ColumnIndex>>\n<output = %<Table>>
  VTQEN_PedalTqSportLoD_pct : Outport
  VTQEN_PedalTqSportlHiD_pct : Outport  Port=2
  wires:
  LookupTable/1 -> VTQEN_PedalTqSportLoD_pct/1  "VTQEN_PedalTqSportLoD_pct"
  LookupTable1/1 -> VTQEN_PedalTqSportlHiD_pct/1  "VTQEN_PedalTqSportlHiD_pct"
  [VDINR_HWAccelPedalPosn_pct] -> LookupTable1/1
  VDINR_EngSpd_erpm/1 -> LookupTable1/2, LookupTable/2
  VDINR_HWAccelPedalPosn_pct/1 -> [VDINR_HWAccelPedalPosn_pct], LookupTable/1

== system tqen/TQEN/PedalTorqueDemand/PedalTorqueDemandCalculation/PedalTorqueCalculation/TqSupport4QuickPedalChange ==
  VDINR_HWAccelPedalPosn_pct : Inport
  task_time_s : Inport  Port=2
  Constant2 : Constant  Value=KTQEN_AccelPedalFiltTm_s
  Constant3 : Constant  Value=ZERO_FLOAT  OutDataTypeStr=single
  FirstOrderFilter : hcu_lib/FirstOrderFilter  SystemSampleTime=-1
  Gain4 : Gain  Gain=4  OutDataTypeStr=single
  IC : UnitDelay  Tag=struct('comment',struct('text','','placement',1),'logdata',struct('maxnumvals',inf,'plotchannels',[],'stepsize',0,'downsampling',1,'loggingmode',3,'channels',1),'output',struct('width',1,'name','$S_$B','unit','','type','Int16','offset',0,'max',NaN,'min',NaN,'freeze',1,'lsb',1,'arb',0,'class','default','address','','description','','autoscalingmode',1,'lowerheadroom',1,'upperheadroom',1,'headroomunit','bit','checkmin',0,'checkmax',0,'show',0,'initial','2'),'state',0,'dt','-1','date',731455.586925799)  SampleTime=-1
  Lookup Table2 : Lookup  InputValues=MTQEN_BaseTqSupptDeltPdlD_X_pctps  Table=MTQEN_BaseTqSupptDeltPdlD_Y_pct  LookUpMeth=Interpolation-Use End Values
      settings: AttributesFormatString=<input =%<InputValues>>\n<output = %<Table>>
  Subtract2 : Sum  Inputs=+-
  Switch1 : Switch  Tag=struct('comment',struct('text','','placement',1),'logdata',struct('maxnumvals',inf,'plotchannels',[],'stepsize',0,'downsampling',1,'loggingmode',3,'channels',1),'output',struct('width',1,'name','$S_$B','unit','','type','Int32Bin15','offset',0,'max',65535,'min',-65536,'freeze',1,'lsb',2^-15,'arb',0,'class','default','address','','description','','autoscalingmode',1,'lowerheadroom',1,'upperheadroom',1,'headroomunit','bit','checkmin',0,'checkmax',0,'show',0),'threshold',struct('width',1,'name','$S_$B_threshold','unit','','type','Int16','offset',0,'max',NaN,'min',NaN,'freeze',1,'lsb',1,'arb',0,'class','default','address','','description','','value','1','scalar',0),'date',731455.58657044)  Threshold=0.5  InputSameDT=on
  Unit Delay{,1..3} (4 alike) : UnitDelay  SampleTime=-1
  lib_divide5 : tqen/lib_divide5
  zero : Constant  Tag=struct('comment',struct('text','','placement',1),'output',struct('width',1,'name','$S_$B','unit','','type','Int16','offset',0,'max',NaN,'min',NaN,'freeze',1,'lsb',1,'arb',0,'class','default','address','','description','','value','0','tolerance',1,'show',0),'date',731455.58675544)  Value=TRUE
  zero1 : Constant  Tag=struct('comment',struct('text','','placement',1),'output',struct('width',1,'name','$S_$B','unit','','type','Int16','offset',0,'max',NaN,'min',NaN,'freeze',1,'lsb',1,'arb',0,'class','default','address','','description','','value','0','tolerance',1,'show',0),'date',731455.58675544)  Value=0  OutDataTypeStr=single
  VTQEN_DeltPedalComp_pct : Outport
  wires:
  Constant2/1 -> Switch1/1
  zero1/1 -> Switch1/3
  IC/1 -> Switch1/2
  zero/1 -> IC/1
  Switch1/1 -> FirstOrderFilter/2
  task_time_s/1 -> FirstOrderFilter/3, Gain4/1
  Unit Delay/1 -> Unit Delay1/1
  Unit Delay1/1 -> Unit Delay2/1
  FirstOrderFilter/1 -> Unit Delay/1, Subtract2/1
  Unit Delay2/1 -> Unit Delay3/1
  Subtract2/1 -> lib_divide5/1
  Gain4/1 -> lib_divide5/2
  Constant3/1 -> lib_divide5/3
  lib_divide5/1 -> Lookup Table2/1
  VDINR_HWAccelPedalPosn_pct/1 -> FirstOrderFilter/1
  Lookup Table2/1 -> VTQEN_DeltPedalComp_pct/1  "VTQEN_DeltPedalComp_pct"
  Unit Delay3/1 -> Subtract2/2

== system tqen/TQEN/CruiseControl/CruiseController/PI Controller for Cruise Control/Integrator/Saturation ==
  in : Inport
  min : Inport  Port=2
  max : Inport  Port=3
  MinMax : MinMax  Function=max  Inputs=2  ZeroCross=off  SaturateOnIntegerOverflow=on  InputSameDT=on
  MinMax1 : MinMax  Inputs=2  ZeroCross=off  SaturateOnIntegerOverflow=on  InputSameDT=on
  out : Outport
  wires:
  MinMax1/1 -> out/1
  max/1 -> MinMax1/2
  min/1 -> MinMax/2
  in/1 -> MinMax/1
  MinMax/1 -> MinMax1/1

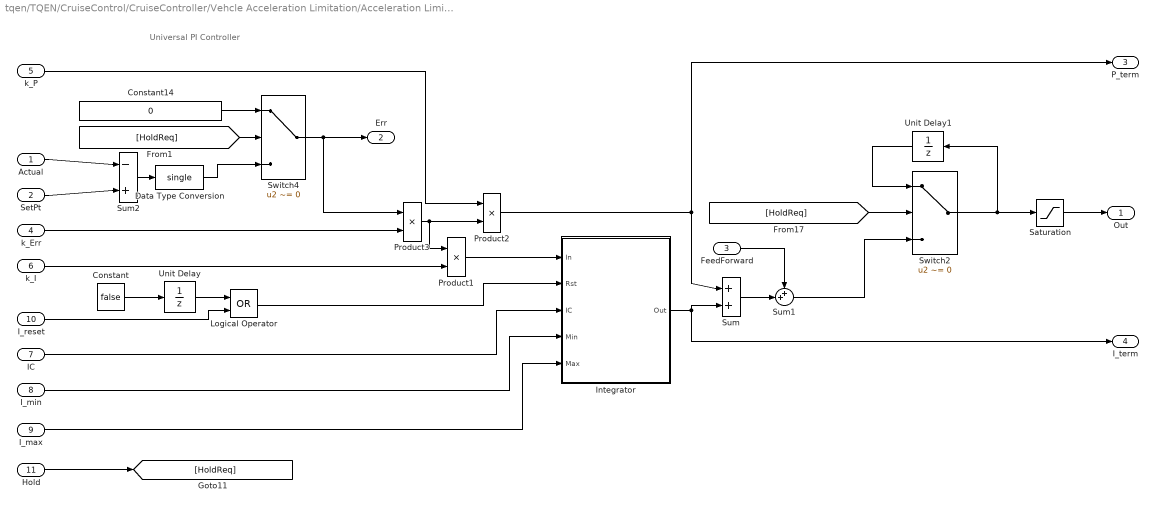
== system tqen/TQEN/CruiseControl/CruiseController/Vehcle Acceleration Limitation/Acceleration Limitation/PI Controller for Acceleration Limiter ==
  note: Universal PI Controller
  Actual : Inport
  SetPt : Inport  Port=2
  FeedForward : Inport  Port=3
  k_Err : Inport  Port=4
  k_P : Inport  Port=5
  k_I : Inport  Port=6
  IC : Inport  Port=7
  I_min : Inport  Port=8
  I_max : Inport  Port=9
  I_reset : Inport  Port=10
  Hold : Inport  Port=11
  Constant : Constant  Value=false  OutDataTypeStr=boolean
  Constant14 : Constant  Value=0  OutDataTypeStr=single
  Data Type Conversion : DataTypeConversion  OutDataTypeStr=single  SaturateOnIntegerOverflow=on  RndMeth=Zero
  Integrator : Subsystem  TreatAsAtomicUnit=on
  Logical Operator : Logic  Operator=OR  AllPortsSameDT=off  OutDataTypeStr=boolean
  Product1 : Product  InputSameDT=on  OutDataTypeStr=Inherit: Same as first input
  Product2 : Product  InputSameDT=on  OutDataTypeStr=Inherit: Same as first input
  Product3 : Product  InputSameDT=on  OutDataTypeStr=Inherit: Same as first input
  Saturation : Saturate  UpperLimit=inf  LowerLimit=0
  Sum : Sum  Inputs=+|+  SaturateOnIntegerOverflow=on  InputSameDT=on  OutDataTypeStr=Inherit: Same as first input
  Sum1 : Sum  Inputs=++|
  Sum2 : Sum  Inputs=-|+  SaturateOnIntegerOverflow=on  InputSameDT=on  OutDataTypeStr=Inherit: Same as first input
  Switch2 : Switch  Criteria=u2 ~= 0
  Switch4 : Switch  Criteria=u2 ~= 0
  Unit Delay : UnitDelay  InitialCondition=true  SampleTime=-1
  Unit Delay1 : UnitDelay  SampleTime=-1
  Out : Outport  OutputWhenDisabled=reset  InitialOutput=[0]
  Err : Outport  Port=2  OutputWhenDisabled=reset  InitialOutput=[0]
  P_term : Outport  Port=3  OutputWhenDisabled=reset  InitialOutput=[0]
  I_term : Outport  Port=4  OutputWhenDisabled=reset  InitialOutput=[0]
  wires:
  I_max/1 -> Integrator/5(Max)
  I_min/1 -> Integrator/4(Min)
  k_Err/1 -> Product3/2
  SetPt/1 -> Sum2/2
  Actual/1 -> Sum2/1
  k_P/1 -> Product2/1
  k_I/1 -> Product1/2
  Product1/1 -> Integrator/1(In)
  Product2/1 -> P_term/1, Sum/1
  Integrator/1(Out) -> I_term/1, Sum/2
  Sum/1 -> Sum1/2
  IC/1 -> Integrator/3(IC)
  Product3/1 -> Product2/2, Product1/1
  Sum2/1 -> Data Type Conversion/1
  Logical Operator/1 -> Integrator/2(Rst)
  I_reset/1 -> Logical Operator/2
  Unit Delay/1 -> Logical Operator/1
  Constant/1 -> Unit Delay/1
  Hold/1 -> [HoldReq]
  [HoldReq] -> Switch2/2
  Switch2/1 -> Unit Delay1/1, Saturation/1
  Unit Delay1/1 -> Switch2/1
  Switch4/1 -> Err/1, Product3/1
  Data Type Conversion/1 -> Switch4/3
  [HoldReq] -> Switch4/2
  Constant14/1 -> Switch4/1
  Sum1/1 -> Switch2/3
  FeedForward/1 -> Sum1/1
  Saturation/1 -> Out/1

== system tqen/TQEN/Governor/Vehcle Speed Governing/Vehicle Speed Governor/PI Controller for Vehicle Governor/Integrator ==
  In : Inport
  Rst : Inport  Port=2
  IC : Inport  Port=3
  Min : Inport  Port=4
  Max : Inport  Port=5
  Constant : Constant  Value=C_TICK_TIME_S  OutDataTypeStr=single
  Data Type Conversion : DataTypeConversion  OutDataTypeStr=boolean  RndMeth=Zero
  Product : Product  SaturateOnIntegerOverflow=on  InputSameDT=on  OutDataTypeStr=Inherit: Same as first input
  Saturation : Subsystem
  Sum : Sum  Inputs=++|  SaturateOnIntegerOverflow=on  InputSameDT=on
  Switch1 : Switch  Threshold=1  ZeroCross=off  SaturateOnIntegerOverflow=on  InputSameDT=on
  Unit Delay : UnitDelay  SampleTime=-1
  Out : Outport
  wires:
  Saturation/1(out) -> Unit Delay/1
  Sum/1 -> Saturation/1(in)
  Switch1/1 -> Out/1, Sum/1
  Constant/1 -> Product/2
  In/1 -> Product/1
  Product/1 -> Sum/2
  Unit Delay/1 -> Switch1/3
  Rst/1 -> Data Type Conversion/1
  Data Type Conversion/1 -> Switch1/2
  Min/1 -> Saturation/2(min)
  Max/1 -> Saturation/3(max)
  IC/1 -> Switch1/1

== system tqen/TQEN/CruiseControl/CruiseController/Vehcle Acceleration Limitation/Acceleration Limitation/PI Controller for Acceleration Limiter/Integrator ==
  In : Inport
  Rst : Inport  Port=2
  IC : Inport  Port=3
  Min : Inport  Port=4
  Max : Inport  Port=5
  Constant : Constant  Value=C_TICK_TIME_S  OutDataTypeStr=single
  Data Type Conversion : DataTypeConversion  OutDataTypeStr=boolean  RndMeth=Zero
  Product : Product  SaturateOnIntegerOverflow=on  InputSameDT=on  OutDataTypeStr=Inherit: Same as first input
  Saturation : Subsystem
  Sum : Sum  Inputs=++|  SaturateOnIntegerOverflow=on  InputSameDT=on
  Switch1 : Switch  Threshold=1  ZeroCross=off  SaturateOnIntegerOverflow=on  InputSameDT=on
  Unit Delay : UnitDelay  SampleTime=-1
  Out : Outport
  wires:
  Saturation/1(out) -> Unit Delay/1
  Sum/1 -> Saturation/1(in)
  Switch1/1 -> Out/1, Sum/1
  Constant/1 -> Product/2
  In/1 -> Product/1
  Product/1 -> Sum/2
  Unit Delay/1 -> Switch1/3
  Rst/1 -> Data Type Conversion/1
  Data Type Conversion/1 -> Switch1/2
  Min/1 -> Saturation/2(min)
  Max/1 -> Saturation/3(max)
  IC/1 -> Switch1/1

== system tqen/TQEN/Governor/Vehcle Speed Governing/Vehicle Speed Governor/PI Controller for Vehicle Governor/Integrator/Saturation ==
  in : Inport
  min : Inport  Port=2
  max : Inport  Port=3
  MinMax : MinMax  Function=max  Inputs=2  ZeroCross=off  SaturateOnIntegerOverflow=on  InputSameDT=on
  MinMax1 : MinMax  Inputs=2  ZeroCross=off  SaturateOnIntegerOverflow=on  InputSameDT=on
  out : Outport
  wires:
  MinMax1/1 -> out/1
  max/1 -> MinMax1/2
  min/1 -> MinMax/2
  in/1 -> MinMax/1
  MinMax/1 -> MinMax1/1

== system tqen/TQEN/CruiseControl/CruiseController/Vehcle Acceleration Limitation/Acceleration Limitation/PI Controller for Acceleration Limiter/Integrator/Saturation ==
  in : Inport
  min : Inport  Port=2
  max : Inport  Port=3
  MinMax : MinMax  Function=max  Inputs=2  ZeroCross=off  SaturateOnIntegerOverflow=on  InputSameDT=on
  MinMax1 : MinMax  Inputs=2  ZeroCross=off  SaturateOnIntegerOverflow=on  InputSameDT=on
  out : Outport
  wires:
  MinMax1/1 -> out/1
  max/1 -> MinMax1/2
  min/1 -> MinMax/2
  in/1 -> MinMax/1
  MinMax/1 -> MinMax1/1

== stateflow chart TQEN/CruiseControl/Cruise Control Enable Determination ==
  state Initialize
    en:VTQEN_CruzStandby_flg=FALSE;
    en:VTQEN_CruzEnblOn_flg=FALSE;
    en:VTQEN_CruzResumeOn_flg=FALSE;
  state StandBy
    en:VTQEN_CruzStandby_flg=TRUE;
    state WaitForSet
      en:VTQEN_CruzEnblOn_flg=FALSE;
      en:VTQEN_CruzResumeOn_flg=FALSE;
    state CruiseSet
      en:VTQEN_CruzEnblOn_flg=TRUE;
      en:VTQEN_CruzResumeOn_flg=FALSE;
    state CruiseRes
      en:VTQEN_CruzEnblOn_flg=TRUE;
      en:VTQEN_CruzResumeOn_flg=TRUE;
    state CruiseInactive
      en:VTQEN_CruzEnblOn_flg=FALSE;
      en:VTQEN_CruzResumeOn_flg=FALSE;
    (default) -> WaitForSet
    WaitForSet -> CruiseSet : [VTQEN_CruzContSetSW_flg && ...
        | !VDINR_BrkLampOn_flg]
    CruiseSet -> CruiseInactive : [VDINR_BrkLampOn_flg]
    CruiseInactive -> CruiseSet [order 1] : [VTQEN_CruzContSetSW_flg && ...
        | !VDINR_BrkLampOn_flg]
    CruiseRes -> CruiseInactive : [VDINR_BrkLampOn_flg]
    CruiseInactive -> CruiseRes [order 2] : [VTQEN_CruzContResumeSW_flg && ...
        | !VDINR_BrkLampOn_flg]
  (default) -> Initialize
  StandBy -> Initialize : [!VTQEN_CruzContEnblSW_flg]
  Initialize -> StandBy : [VTQEN_CruzContEnblSW_flg]
  data: VTQEN_CruzStandby_flg output double; VDINR_BrkLampOn_flg input double; VTQEN_CruzEnblOn_flg output double; VTQEN_CruzContEnblSW_flg input double; VTQEN_CruzContSetSW_flg input double; VTQEN_CruzContResumeSW_flg input double; VTQEN_CruzResumeOn_flg output double; TRUE parameter double; FALSE parameter double

== stateflow chart TQEN/CruiseControl/Rate_Limit/RateLimiter/Chart ==
  state Increase
    en:
    tou=increase_tou;
    Max=Data_in;
    Min=-10000000000;
    Initial=0;
    du:
    tou=increase_tou;
    Max=Data_in;
    Min=-10000000000;
    Initial=0;
  state Decrease
    en:
    tou=decrease_tou;
    Max=10000000000;
    Min=Data_in;
    Initial=0;
    du:
    tou=decrease_tou;
    Max=10000000000;
    Min=Data_in;
    Initial=0;
  state Start
    en:
    tou=0;
    Max=10000000000;
    Min=-10000000000;
    Initial=1;
  (default) -> Start
  Start -> Increase [order 2] : [increase]
  Start -> Decrease [order 1] : [decrease]
  Increase -> Decrease : [decrease]
  Decrease -> Increase : [increase]
  data: Initial output single; increase input double; decrease input double; Data_in input double; increase_tou input double; decrease_tou input double; tou output single; Min output single; Max output single

== stateflow chart TQEN/CruiseControl/Set Speed Determination ==
  state Initialize
    en:VTQEN_CruzSetSpd_kph=0;
    en:VTQEN_CruzSetSpdIni_kph=0;
    en:CurrSetSpd=VDINR_VehSpd_kph;
  state CruiseEnable
    state SetOn
      en:VTQEN_CruzSetSpd_kph=VDINR_VehSpd_kph;
      en:VTQEN_CruzSetSpdIni_kph=VDINR_VehSpd_kph;
      en:CurrSetSpd=VDINR_VehSpd_kph;
    state ResOn
      en:VTQEN_CruzSetSpd_kph=VTQEN_CruzSetSpdLast_kph;
      en:VTQEN_CruzSetSpdIni_kph=VTQEN_CruzSetSpdLast_kph;
      en:CurrSetSpd=VTQEN_CruzSetSpdLast_kph;
    state WaitingForSpdChange
      en:VTQEN_CruzSetSpd_kph=CurrSetSpd;
      en:VTQEN_CruzSetSpdIni_kph=CurrSetSpd;
    state PrepareToInc
    state PrepareToDec
    state Increase1
      ex: CurrSetSpd=CurrSetSpd+1;
    state Increase10
      ex: CurrSetSpd=CurrSetSpd+10;
    state Decrease1
      ex: CurrSetSpd=CurrSetSpd-1;
    state Decrease10
      ex: CurrSetSpd=CurrSetSpd-10;
    (default) -> (junction 60)
    (junction 60) -> ResOn [order 1] : [VTQEN_CruzResumeOn_flg]
    (junction 60) -> SetOn [order 2] : [!VTQEN_CruzResumeOn_flg]
    ResOn -> WaitingForSpdChange : [!VTQEN_CruzContSetSW_flg &&...
        | !VTQEN_CruzContResumeSW_flg]
    SetOn -> WaitingForSpdChange : [!VTQEN_CruzContSetSW_flg &&...
        | !VTQEN_CruzContResumeSW_flg]
    Increase10 -> WaitingForSpdChange
    Increase1 -> WaitingForSpdChange
    WaitingForSpdChange -> PrepareToInc [order 2] : [VTQEN_CruzContResumeSW_flg]
    (junction 62) -> WaitingForSpdChange [order 3]
    WaitingForSpdChange -> PrepareToDec [order 1] : [VTQEN_CruzContSetSW_flg]
    (junction 61) -> WaitingForSpdChange [order 2]
    Decrease10 -> WaitingForSpdChange
    Decrease1 -> WaitingForSpdChange
    PrepareToDec -> (junction 62) [order 1] : after(VTQEN_CruzSpdChgTimeThres_s/C_TICK_TIME_S,tick) ...
        | [!VTQEN_CruzContSetSW_flg]
    PrepareToInc -> Increase10 [order 1] : after(VTQEN_CruzSpdChgTimeThres_s/C_TICK_TIME_S,tick)...
        | [!VTQEN_CruzContResumeSW_flg]
    PrepareToDec -> (junction 61) [order 2] : [!VTQEN_CruzContSetSW_flg]
    PrepareToInc -> Increase1 [order 2] : [!VTQEN_CruzContResumeSW_flg]
    (junction 61) -> Decrease1 [order 1] : [CurrSetSpd>=1]
    (junction 62) -> Decrease1 [order 1] : [CurrSetSpd>=1 && ...
        |  CurrSetSpd<10]
    (junction 62) -> Decrease10 [order 2] : [CurrSetSpd>=10]
  state Inactive
    en:VTQEN_CruzSetSpd_kph=0;
  (default) -> Initialize
  Initialize -> CruiseEnable : [VTQEN_CruzEnblOn_flg]
  Inactive -> CruiseEnable : [VTQEN_CruzEnblOn_flg]
  CruiseEnable -> Inactive : [!VTQEN_CruzEnblOn_flg]
  data: VTQEN_CruzEnblOn_flg input double; VTQEN_CruzResumeOn_flg input double; VTQEN_CruzSetSpd_kph output double; VDINR_VehSpd_kph input double; VTQEN_CruzContSetSW_flg input double; VTQEN_CruzContResumeSW_flg input double; VTQEN_CruzSpdChgTimeThres_s input double; VTQEN_CruzSetSpdIni_kph output single; VTQEN_CruzSetSpdLast_kph input double; CurrSetSpd local single; C_TICK_TIME_S parameter double

== stateflow chart TQEN/Governor/Vehcle Speed Governing/Governing State Determination ==
  state VSGOVDisable
    en:VTQEN_VSGOVOn_flg=FALSE;
  state VSGOVEnable
    en:VTQEN_VSGOVOn_flg=TRUE;
  state Start
    en:VTQEN_VSGOVOn_flg=FALSE;
  (default) -> Start
  Start -> VSGOVEnable : [VDINR_VehSpd_kph>VTQEN_VehSpdLimVal_kph]
  VSGOVDisable -> VSGOVEnable : [VDINR_VehSpd_kph>VTQEN_VehSpdLimVal_kph]
  VSGOVEnable -> VSGOVDisable : [VDINR_VehSpd_kph<VTQEN_VehSpdLimVal_kph && ...
      | VTQEN_EngTqSource_enum~=ENUM_ECMTQSOURCE_TORQUELIM]
  data: VTQEN_VehSpdLimVal_kph input double; VDINR_VehSpd_kph input double; VTQEN_EngTqSource_enum input double; VTQEN_VSGOVOn_flg output double; ENUM_ECMTQSOURCE_TORQUELIM parameter double; TRUE parameter double; FALSE parameter double
